simulink model "testModel"  (R2018b)
settings: Solver=VariableStepAuto  StartTime=0.0  StopTime=0  RelTol=1e-3
undefined symbols (not defined in the file or in its folder): liftingBody
settings Model: Creator=mcobb  LastModifiedBy=mcobb

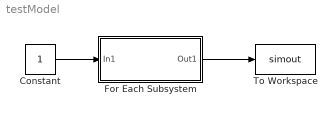
== system testModel ==
  Constant : Constant
  For Each Subsystem : Subsystem  TreatAsAtomicUnit=on  mask{x=liftingBody.forLoopStruct}
  To Workspace : ToWorkspace  VariableName=simout  SaveFormat=Timeseries  SampleTime=-1
  wires:
  Constant/1 -> For Each Subsystem/1(In1)
  For Each Subsystem/1(Out1) -> To Workspace/1

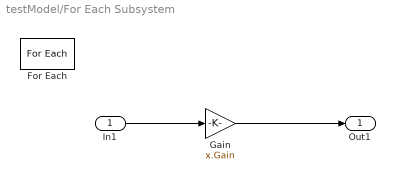
== system testModel/For Each Subsystem ==
  In1 : Inport
  For Each : ForEach  DisableCoverage=on  IterateSubsysMaskParameter=on  SubsysMaskParameterIterationDimension=2  IndexMode=One-based
  Gain : Gain  Gain=x.Gain
  Out1 : Outport  ConcatenationDimension=1
  wires:
  In1/1 -> Gain/1
  Gain/1 -> Out1/1
